simulink model "lindraw"  (R2015a)
settings: Solver=ode45  StartTime=0.0  StopTime=10.0  RelTol=1e-3
values from neighbouring files (symbols this model uses):
  K = place(A,B',p)    [discretizareN.m]    (also in statefb.m = place(A2,B2',p))
  Kd = place(Ad,Bd',p)    [discretizare.m]    (also in discretizareL.m = place(Ad,Bd,p); statefb.m)
settings Model: Creator=asus  LastModifiedBy=asus

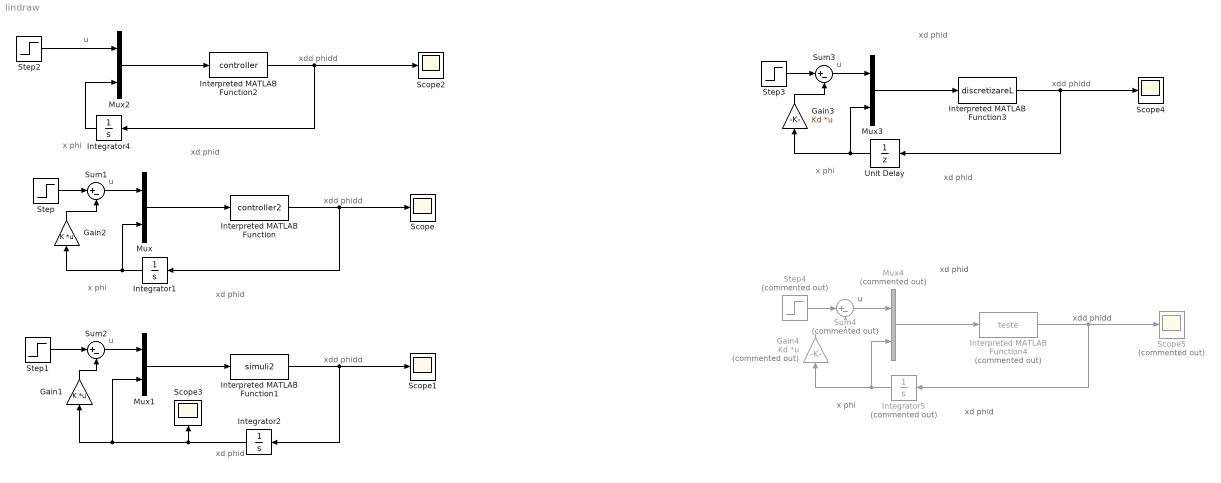
== system lindraw ==
  note: x phi
  note: xd phid
  note: xdd phidd
  note: u
  note: x phi
  note: xd phid
  note: xdd phidd
  note: u
  note: xd phid
  note: xdd phidd
  note: u
  note: x phi
  note: xd phid
  note: xdd phidd
  note: u
  note: xd phid
  note: x phi
  note: xd phid
  note: xdd phidd
  note: u
  note: xd phid
  Gain1 : Gain  Gain=K  Multiplication=Matrix(K*u) (u vector)
  Gain2 : Gain  Gain=K  Multiplication=Matrix(K*u) (u vector)
  Gain3 : Gain  Gain=Kd  Multiplication=Matrix(K*u) (u vector)
  Gain4 : Gain  Commented=on  Gain=Kd  Multiplication=Matrix(K*u) (u vector)
  Integrator1 : Integrator  InitialCondition=[0;1;1;2]
  Integrator2 : Integrator  InitialCondition=[1;2;3;3]
  Integrator4 : Integrator  InitialCondition=[0;1;1;2]
  Integrator5 : Integrator  Commented=on  InitialCondition=[0;1;1;2]
  Interpreted MATLAB Function : MATLABFcn  MATLABFcn=controller2
  Interpreted MATLAB Function1 : MATLABFcn  MATLABFcn=simuli2
  Interpreted MATLAB Function2 : MATLABFcn  MATLABFcn=controller
  Interpreted MATLAB Function3 : MATLABFcn  MATLABFcn=discretizareL
  Interpreted MATLAB Function4 : MATLABFcn  Commented=on  MATLABFcn=teste
  Mux{,1..3} (4 alike) : Mux  Inputs=2
  Mux4 : Mux  Commented=on  Inputs=2
  Scope{,1..4} (5 alike) : Scope
      Scope settings: YMin=-0.225  YMax=0.2
      Scope1 settings: YMin=-5e+07  YMax=4.5e+08
      Scope2 settings: SaveName=ScopeData2
      Scope3 settings: YMin=-250000  YMax=3.75e+06  SaveName=ScopeData3
      Scope4 settings: YMin=-0.225  YMax=0.2  SaveName=ScopeData4
  Scope5 : Scope  Commented=on
      settings: YMin=-0.225  YMax=0.2  SaveName=ScopeData5
  Step : Step  Time=0  After=0  SampleTime=0
  Step1 : Step  Time=0  After=0  SampleTime=0  ZeroCross=off
  Step2 : Step  Time=0  After=0  SampleTime=0
  Step3 : Step  Time=0  After=0  SampleTime=0
  Step4 : Step  Commented=on  Time=0  After=0  SampleTime=0
  Sum1 : Sum  Inputs=|+-
  Sum2 : Sum  Inputs=|+-
  Sum3 : Sum  Inputs=|+-
  Sum4 : Sum  Commented=on  Inputs=|+-
  Unit Delay : UnitDelay  InitialCondition=[0;1;1;2]  SampleTime=-1
  wires:
  Mux/1 -> Interpreted MATLAB Function/1
  Interpreted MATLAB Function/1 -> Integrator1/1, Scope/1
  Integrator1/1 -> Gain2/1, Mux/2
  Step/1 -> Sum1/1
  Gain2/1 -> Sum1/2
  Sum1/1 -> Mux/1
  Mux2/1 -> Interpreted MATLAB Function2/1
  Interpreted MATLAB Function2/1 -> Scope2/1, Integrator4/1
  Integrator4/1 -> Mux2/2
  Step2/1 -> Mux2/1
  Mux1/1 -> Interpreted MATLAB Function1/1
  Interpreted MATLAB Function1/1 -> Integrator2/1, Scope1/1
  Step1/1 -> Sum2/1
  Gain1/1 -> Sum2/2
  Sum2/1 -> Mux1/1
  Integrator2/1 -> Scope3/1, Mux1/2, Gain1/1
  Mux3/1 -> Interpreted MATLAB Function3/1
  Interpreted MATLAB Function3/1 -> Unit Delay/1, Scope4/1
  Unit Delay/1 -> Gain3/1, Mux3/2
  Step3/1 -> Sum3/1
  Gain3/1 -> Sum3/2
  Sum3/1 -> Mux3/1
  Mux4/1 -> Interpreted MATLAB Function4/1
  Interpreted MATLAB Function4/1 -> Integrator5/1, Scope5/1
  Integrator5/1 -> Gain4/1, Mux4/2
  Step4/1 -> Sum4/1
  Gain4/1 -> Sum4/2
  Sum4/1 -> Mux4/1
